simulink model "test02"  (R2021a)
settings: Solver=VariableStepAuto  StartTime=0.0  StopTime=10.0  RelTol=1e-3
libraries: spsDiodeLib x6, spsSeriesRLCBranchLib x6, spsIdealSwitchLib x6, spsThyristorLib x6, spsVoltageMeasurementLib x6, spsDCVoltageSourceLib x2, spspowerguiLib x1
settings Model: Creator=shashank  LastModifiedBy=shashank

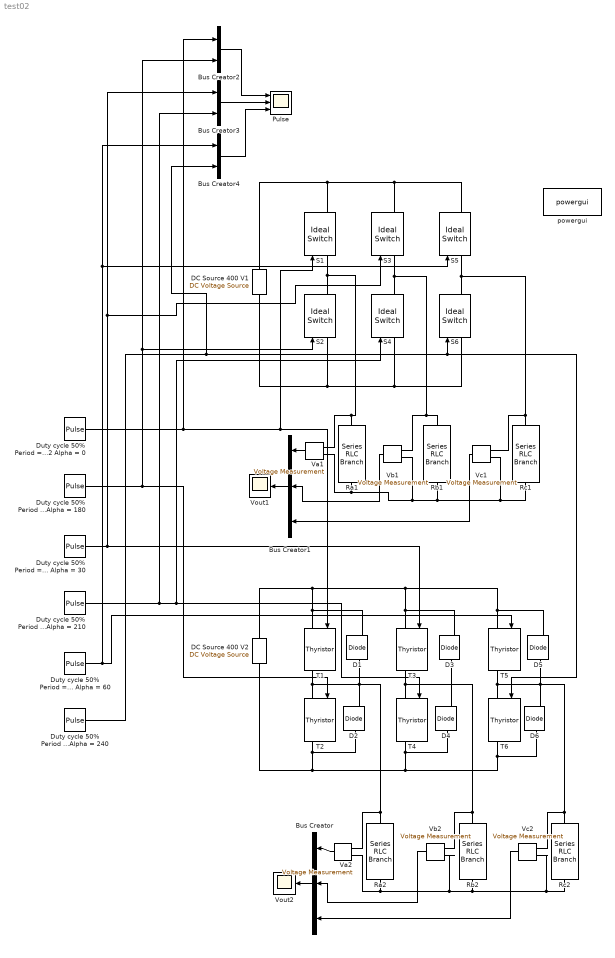
== system test02 ==
  Bus Creator : BusCreator  Inputs=3
  Bus Creator1 : BusCreator  Inputs=3
  Bus Creator2 : BusCreator  Inputs=2
  Bus Creator3 : BusCreator  Inputs=2
  Bus Creator4 : BusCreator  Inputs=2
  D{1..6} (6 alike) : spsDiodeLib/Diode  Ron=0.001  Lon=0  Vf=0.8  IC=0  UseSnubber=0  Rs=500  Cs=250e-9  Measurements=on
  DC Source 400 V1 : spsDCVoltageSourceLib/DC Voltage Source  Amplitude=400  Measurements=Voltage
  DC Source 400 V2 : spsDCVoltageSourceLib/DC Voltage Source  Amplitude=400  Measurements=None
  Duty cycle 50% Period = 0.02 Alpha = 0 : DiscretePulseGenerator  PulseType=Time based  Period=1/50  PulseWidth=50  PhaseDelay=(0.02/360) * 0
  Duty cycle 50% Period = 0.02 Alpha = 180 : DiscretePulseGenerator  PulseType=Time based  Period=1/50  PulseWidth=50  PhaseDelay=(0.02/360) * 180
  Duty cycle 50% Period = 0.02 Alpha = 210 : DiscretePulseGenerator  PulseType=Time based  Period=1/50  PulseWidth=50  PhaseDelay=(0.02/360) * 210
  Duty cycle 50% Period = 0.02 Alpha = 240 : DiscretePulseGenerator  PulseType=Time based  Period=1/50  PulseWidth=50  PhaseDelay=(0.02/360) * 240
  Duty cycle 50% Period = 0.02 Alpha = 30 : DiscretePulseGenerator  PulseType=Time based  Period=1/50  PulseWidth=50  PhaseDelay=(0.02/360) * 30
  Duty cycle 50% Period = 0.02 Alpha = 60 : DiscretePulseGenerator  PulseType=Time based  Period=1/50  PulseWidth=50  PhaseDelay=(0.02/360) * 60
  Pulse : Scope  NumInputPorts=3
  Ra1 : spsSeriesRLCBranchLib/Series RLC Branch  LConnTagsString=__new0  RConnTagsString=__new0  BranchType=R  Resistance=10  Inductance=1e-3  SetiL0=off  InitialCurrent=0  Capacitance=1e-6  Setx0=off  InitialVoltage=0  Measurements=None
  Ra2 : spsSeriesRLCBranchLib/Series RLC Branch  LConnTagsString=__new0  RConnTagsString=__new0  BranchType=R  Resistance=10  Inductance=1e-3  SetiL0=off  InitialCurrent=0  Capacitance=1e-6  Setx0=off  InitialVoltage=0  Measurements=None
  Rb1 : spsSeriesRLCBranchLib/Series RLC Branch  LConnTagsString=__new0  RConnTagsString=__new0  BranchType=R  Resistance=10  Inductance=1e-3  SetiL0=off  InitialCurrent=0  Capacitance=1e-6  Setx0=off  InitialVoltage=0  Measurements=None
  Rb2 : spsSeriesRLCBranchLib/Series RLC Branch  LConnTagsString=__new0  RConnTagsString=__new0  BranchType=R  Resistance=10  Inductance=1e-3  SetiL0=off  InitialCurrent=0  Capacitance=1e-6  Setx0=off  InitialVoltage=0  Measurements=None
  Rc1 : spsSeriesRLCBranchLib/Series RLC Branch  LConnTagsString=__new0  RConnTagsString=__new0  BranchType=R  Resistance=10  Inductance=1e-3  SetiL0=off  InitialCurrent=0  Capacitance=1e-6  Setx0=off  InitialVoltage=0  Measurements=None
  Rc2 : spsSeriesRLCBranchLib/Series RLC Branch  LConnTagsString=__new0  RConnTagsString=__new0  BranchType=R  Resistance=10  Inductance=1e-3  SetiL0=off  InitialCurrent=0  Capacitance=1e-6  Setx0=off  InitialVoltage=0  Measurements=None
  S{1..6} (6 alike) : spsIdealSwitchLib/Ideal Switch  Ron=0.001  Lon=0  IC=0  Rs=1e5  Cs=inf  Measurements=on
  T{1..6} (6 alike) : spsThyristorLib/Thyristor  Ron=0.001  Lon=0  Vf=0.8  IC=0  Rs=500  Cs=250e-9  Measurements=on
  Va1 : spsVoltageMeasurementLib/Voltage Measurement  PhasorSimulation=off  OutputType=Complex  PSBequivalent=0
  Va2 : spsVoltageMeasurementLib/Voltage Measurement  PhasorSimulation=off  OutputType=Complex  PSBequivalent=0
  Vb1 : spsVoltageMeasurementLib/Voltage Measurement  PhasorSimulation=off  OutputType=Complex  PSBequivalent=0
  Vb2 : spsVoltageMeasurementLib/Voltage Measurement  PhasorSimulation=off  OutputType=Complex  PSBequivalent=0
  Vc1 : spsVoltageMeasurementLib/Voltage Measurement  PhasorSimulation=off  OutputType=Complex  PSBequivalent=0
  Vc2 : spsVoltageMeasurementLib/Voltage Measurement  PhasorSimulation=off  OutputType=Complex  PSBequivalent=0
  Vout1 : Scope
  Vout2 : Scope
  powergui : spspowerguiLib/powergui  Priority=1  SimulationMode=Continuous  SampleTime=50e-6  frequency=60  Iterations=50  frequencyindice=0  Pbase=100e6  ErrMax=1e-4  UnitsV=kV  UnitsW=MW  buscounter=0  FunctionMessages=off  echomessages=off  EnableUseOfTLC=off  CurrentSourceSwitches=off  DisableSnubberDevices=off  DisableRonSwitches=off  DisableVfSwitches=off  DisplayEquations=off  AutomaticDiscreteSolvers=off  SolverType=Tustin/Backward Euler (TBE)  Interpol=off  ExternalGateDelay=off  methode=off  Ts=100  x0status=blocks  SPID=on  SwTol=0  HookPort=off  NonlinearTolerance=1e-4  nMaxIteration=100  ContinueOnMaxIteration=off  RestoreLinks=warning  ResistiveCurrentMeasurement=off  Frange=[0:2:500]  Ylog=off  Xlog=on  ShowGrid=off  save=off  variable=ZData  structure=0  ZoomFFT=off  StartTime=0.0  cycles=1  DisplayStyle=1  fundamental=60  FreqAxis=off  MaxFrequency=1000  frequencyindicesteady=1  RmsSteady=1  display=off
  wires:
  Va2/1 -> Bus Creator/1
  Vb2/1 -> Bus Creator/2
  Vc2/1 -> Bus Creator/3
  Bus Creator/1 -> Vout2/1
  Vc1/1 -> Bus Creator1/3
  Va1/1 -> Bus Creator1/1
  Bus Creator1/1 -> Vout1/1
  Vb1/1 -> Bus Creator1/2
  Duty cycle 50% Period = 0.02 Alpha = 0/1 -> T1/1, S1/1, Bus Creator2/1
  Duty cycle 50% Period = 0.02 Alpha = 180/1 -> S2/1, Bus Creator2/2, T2/1
  Duty cycle 50% Period = 0.02 Alpha = 30/1 -> S3/1, Bus Creator3/1, T3/1
  Duty cycle 50% Period = 0.02 Alpha = 210/1 -> T4/1, S4/1, Bus Creator3/2
  Duty cycle 50% Period = 0.02 Alpha = 60/1 -> S5/1, Bus Creator4/1, T5/1
  Duty cycle 50% Period = 0.02 Alpha = 240/1 -> Bus Creator4/2, T6/1, S6/1
  Bus Creator2/1 -> Pulse/1
  Bus Creator3/1 -> Pulse/2
  Bus Creator4/1 -> Pulse/3
  connections:
  T5/LConn1 -- D5/RConn1 -- D3/RConn1 -- T3/LConn1 -- DC Source 400 V2/RConn1 -- D1/RConn1 -- T1/LConn1
  T6/RConn1 -- D4/LConn1 -- T4/RConn1 -- DC Source 400 V2/LConn1 -- D2/LConn1 -- T2/RConn1 -- D6/LConn1
  T2/LConn1 -- Va2/LConn2 -- Ra2/RConn1 -- D2/RConn1 -- D1/LConn1 -- T1/RConn1
  T4/LConn1 -- Vb2/LConn2 -- Rb2/RConn1 -- T3/RConn1
  T6/LConn1 -- Vc2/LConn2 -- Rc2/RConn1 -- D6/RConn1 -- D5/LConn1 -- T5/RConn1
  D4/RConn1 -- D3/LConn1
  S6/LConn1 -- S4/LConn1 -- DC Source 400 V1/LConn1 -- S2/LConn1
  DC Source 400 V1/RConn1 -- S3/RConn1 -- S5/RConn1 -- S1/RConn1
  Rc1/RConn1 -- S5/LConn1 -- S6/RConn1 -- Vc1/LConn2
  Ra1/RConn1 -- S1/LConn1 -- S2/RConn1 -- Va1/LConn2
  Rb1/RConn1 -- Vb1/LConn2 -- S3/LConn1 -- S4/RConn1
  Vb1/LConn1 -- Vc1/LConn1 -- Rc1/LConn1 -- Rb1/LConn1 -- Va1/LConn1 -- Ra1/LConn1
  Vb2/LConn1 -- Va2/LConn1 -- Ra2/LConn1 -- Rb2/LConn1 -- Vc2/LConn1 -- Rc2/LConn1
